simulink model "partC"  (R2018b)
settings: Solver=VariableStepAuto  StartTime=0.0  StopTime=10.0  RelTol=1e-3
settings Model: Creator=shins  LastModifiedBy=shins

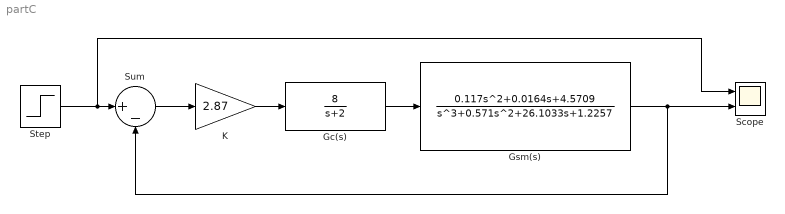
== system partC ==
  Gc(s) : TransferFcn  Numerator=[8]  Denominator=[1 2]
  Gsm(s) : TransferFcn  Numerator=[0.117 0.0164 4.5709]  Denominator=[1 0.571 26.1033 1.2257]
  K : Gain  Gain=2.87
  Scope : Scope  NumInputPorts=2
  Step : Step  Time=0  Before=1  SampleTime=0
  Sum : Sum  Inputs=|+-
  wires:
  Step/1 -> Scope/1, Sum/1
  Sum/1 -> K/1
  K/1 -> Gc(s)/1
  Gc(s)/1 -> Gsm(s)/1
  Gsm(s)/1 -> Sum/2, Scope/2
